simulink model "CONTRO~1"  (R2019a)
settings: Solver=VariableStepAuto  StartTime=0.0  StopTime=10  RelTol=1e-3
values from neighbouring files (symbols this model uses):
  A = [0 1 0;0 0 1;0 -2 -3]    [Controlador1_com_perturbacoes_planta_com_integrador.m]    (also in Controlador1_com_perturbacoes_planta_sem_integrador.m = [0 1 0;0 0 1;-6 -11 -6]; Q2_PCEEP2.m = [0 1 0; 0 0 1; 0 -200 -30]; Q3_PCEEP2.m = [0 1; -8 -4])
  a = [0 1 0;0 0 1;0 -20 -3]    [Controlador1_com_perturbacoes_planta_com_integrador.m]    (also in Controlador1_com_perturbacoes_planta_sem_integrador.m = [0 1 0;0 0 1;-60 -11 -6])
  B = [0 0 1]'    [Controlador1_com_perturbacoes_planta_com_integrador.m]    (also in Controlador1_com_perturbacoes_planta_sem_integrador.m; Q2_PCEEP2.m = [0; 0; 1]; Q3_PCEEP2.m = [0; 1])
  K = acker(A,B,polosMF)    [Controlador1_com_perturbacoes_planta_com_integrador.m]    (also in Controlador1_com_perturbacoes_planta_sem_integrador.m; Q2_PCEEP2.m = acker(A, B, polos_desejados); Q3_PCEEP2.m = acker(A, B, polos_desejados))
settings Model: Creator=rcard  LastModifiedBy=rcard

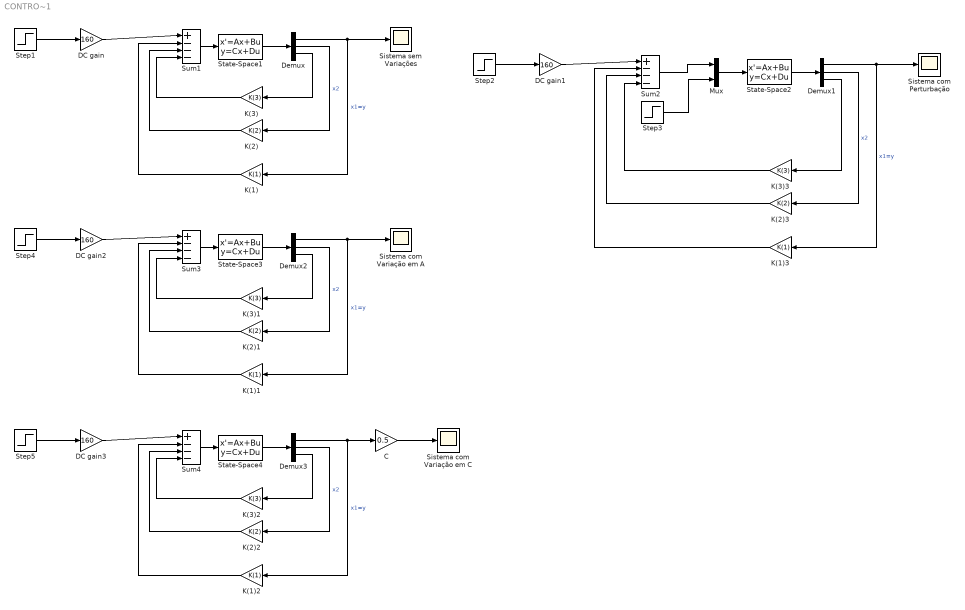
== system CONTRO~1 ==
  C : Gain  Gain=0.5
  DC gain{,1..3} (4 alike) : Gain  Gain=160
  Demux{,1..3} (4 alike) : Demux  Outputs=3
  K(1){,1..3} (4 alike) : Gain  Gain=K(1)
  K(2){,1..3} (4 alike) : Gain  Gain=K(2)
  K(3){,1..3} (4 alike) : Gain  Gain=K(3)
  Mux : Mux  Inputs=2
  "Sistema com Perturbação " : Scope
  Sistema com Variação em A : Scope
  Sistema com Variação em C : Scope
  Sistema sem Variações : Scope
  State-Space1 : StateSpace  A=A  B=B  C=eye(3)  D=zeros(3,1)  InitialCondition=[0 0 0]
  State-Space2 : StateSpace  A=A  B=[B -B]  C=eye(3)  D=zeros(3,2)  InitialCondition=[0 0 0]
  State-Space3 : StateSpace  A=a  B=B  C=eye(3)  D=zeros(3,1)  InitialCondition=[0 0 0]
  State-Space4 : StateSpace  A=A  B=B  C=eye(3)  D=zeros(3,1)  InitialCondition=[0 0 0]
  Step{1..2,4..5} (4 alike) : Step  Time=0  SampleTime=1/20000
  Step3 : Step  Time=5  After=5  SampleTime=1/20000
  Sum{1..4} (4 alike) : Sum  Inputs=|+---
  wires:
  Sum1/1 -> State-Space1/1
  Step1/1 -> DC gain/1
  State-Space1/1 -> Demux/1
  Demux/1 -> K(1)/1, Sistema sem Variações/1  "x1=y"
  Demux/2 -> K(2)/1  "x2"
  K(2)/1 -> Sum1/3
  K(1)/1 -> Sum1/2
  Demux/3 -> K(3)/1
  K(3)/1 -> Sum1/4
  DC gain/1 -> Sum1/1
  DC gain1/1 -> Sum2/1
  Step2/1 -> DC gain1/1
  K(2)3/1 -> Sum2/3
  State-Space2/1 -> Demux1/1
  Demux1/2 -> K(2)3/1  "x2"
  K(3)3/1 -> Sum2/4
  Demux1/3 -> K(3)3/1
  K(1)3/1 -> Sum2/2
  Demux1/1 -> K(1)3/1, "Sistema com Perturbação "/1  "x1=y"
  Mux/1 -> State-Space2/1
  Sum2/1 -> Mux/1
  Step3/1 -> Mux/2
  Demux2/1 -> K(1)1/1, Sistema com Variação em A/1  "x1=y"
  State-Space3/1 -> Demux2/1
  DC gain2/1 -> Sum3/1
  K(3)1/1 -> Sum3/4
  Step4/1 -> DC gain2/1
  Demux2/3 -> K(3)1/1
  Sum3/1 -> State-Space3/1
  K(2)1/1 -> Sum3/3
  Demux2/2 -> K(2)1/1  "x2"
  K(1)1/1 -> Sum3/2
  K(1)2/1 -> Sum4/2
  Demux3/2 -> K(2)2/1  "x2"
  Demux3/3 -> K(3)2/1
  Sum4/1 -> State-Space4/1
  K(3)2/1 -> Sum4/4
  K(2)2/1 -> Sum4/3
  State-Space4/1 -> Demux3/1
  Demux3/1 -> C/1, K(1)2/1  "x1=y"
  DC gain3/1 -> Sum4/1
  Step5/1 -> DC gain3/1
  C/1 -> Sistema com Variação em C/1
